simulink model "Loudspeaker"  (R2023b)
settings: Solver=VariableStepAuto  StartTime=0.0  StopTime=5  RelTol=1e-3
settings Model: Creator=Nishanth S  LastModifiedBy=Nishanth S

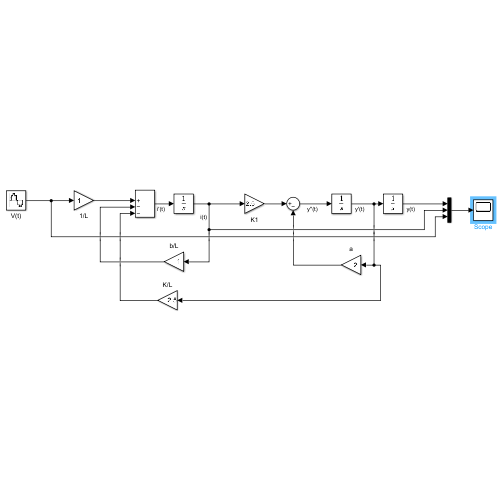
[thumbnail: Simulink's stored preview of the top-level diagram]
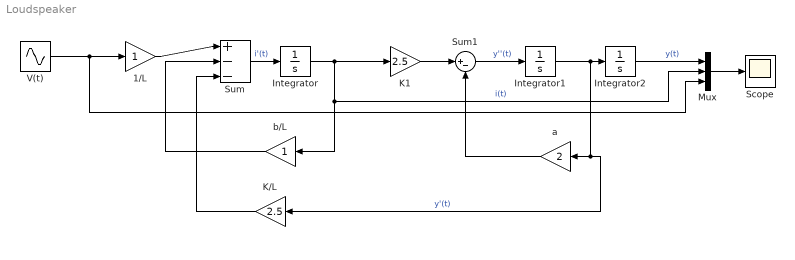
== system Loudspeaker ==
  1/L : Gain
  Integrator : Integrator
  Integrator1 : Integrator
  Integrator2 : Integrator
  K/L : Gain  Gain=2.5
  K1 : Gain  Gain=2.5
  Mux : Mux  Inputs=3
  Scope : Scope
  Sum : Sum  Inputs=|+--
  Sum1 : Sum  Inputs=|+-
  V(t) : Sin  Amplitude=2  Frequency=5  SampleTime=0.001
  a : Gain  Gain=2
  b/L : Gain
  wires:
  Sum/1 -> Integrator/1  "i'(t)"
  Integrator/1 -> b/L/1, Mux/2, K1/1  "i(t)"
  1/L/1 -> Sum/1
  b/L/1 -> Sum/2
  K1/1 -> Sum1/1
  a/1 -> Sum1/2
  Sum1/1 -> Integrator1/1  "y''(t)"
  Integrator1/1 -> K/L/1, a/1, Integrator2/1  "y'(t)"
  Integrator2/1 -> Mux/1  "y(t)"
  K/L/1 -> Sum/3
  Mux/1 -> Scope/1
  V(t)/1 -> 1/L/1, Mux/3
